simulink model "PlantaMalhaExterna_teste"  (R2018b)
settings: Solver=VariableStepAuto  StartTime=0.0  StopTime=10.0  RelTol=1e-3
undefined symbols (not defined in the file or in its folder): DiscIntNeverNeededParam
libraries: simulink x1
settings Model: Creator=lucas  LastModifiedBy=vitor
settings DataIOCC: ReturnWorkspaceOutputs=on
settings DebuggingCC: SFMachineParentedDataDiag=error

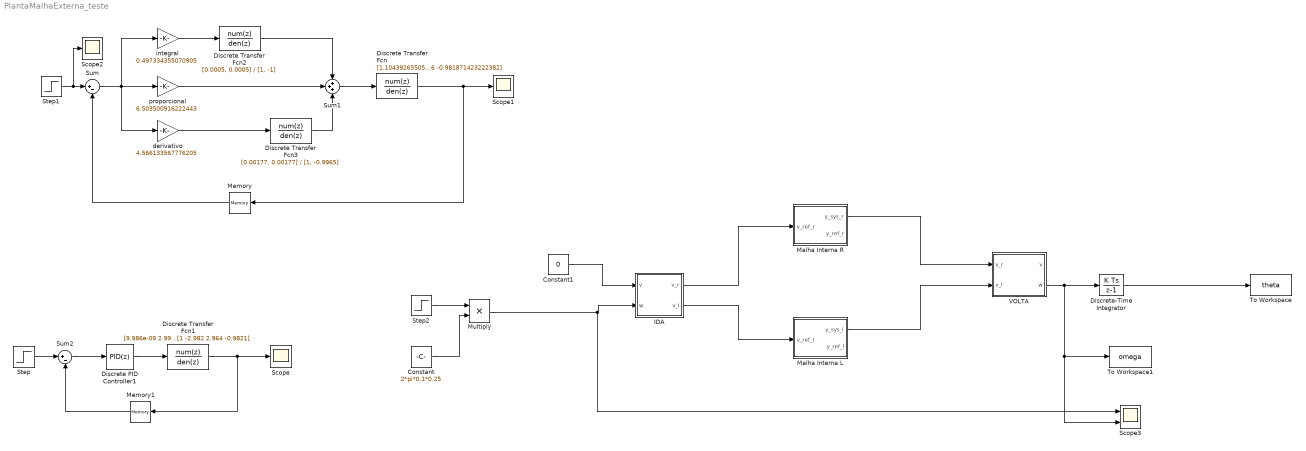
== system PlantaMalhaExterna_teste ==
  Constant : Constant  Value=2*pi*0.1*0.25
  Constant1 : Constant  Value=0
  Discrete Transfer Fcn : DiscreteTransferFcn  Numerator=[1.104392655054829e-08 3.313177965164485e-08 3.313177965164485e-08 1.104392655054829e-08]  Denominator=[1 -2.981694681338594 2.963566104560976 -0.981871423222382]  SampleTime=0.001
  Discrete Transfer Fcn1 : DiscreteTransferFcn  Numerator=[9.986e-09 2.996e-08 2.996e-08 9.986e-09]  Denominator=[1 -2.982 2.964 -0.9821]  SampleTime=0.001
  Discrete Transfer Fcn2 : DiscreteTransferFcn  Numerator=[0.0005, 0.0005]  Denominator=[1, -1]
  Discrete Transfer Fcn3 : DiscreteTransferFcn  Numerator=[0.00177, 0.00177]  Denominator=[1, -0.9965]  SampleTime=0.001
  Discrete PID Controller1 : simulink/Continuous/PID Controller  Controller=PID  Form=Parallel  TimeDomain=Discrete-time  SampleTime=0.001  IntegratorMethod=Forward Euler  FilterMethod=Forward Euler  ControllerParametersSource=internal  P=200  I=0  D=8  UseFilter=on  N=1.824  TunerSelectOption=Transfer Function Based (PID Tuner App)  InitialConditionSource=internal  InitialConditionForIntegrator=0  InitialConditionForFilter=0  DifferentiatorICPrevScaledInput=0  ExternalReset=none  TrackingMode=off  Kt=1  LimitOutput=off  UpperSaturationLimit=inf  LowerSaturationLimit=-inf  LinearizeAsGain=off  AntiWindupMode=none  Kb=1  POutMin=[]  POutMax=[]  IOutMin=[]  IOutMax=[]  DOutMin=[]  DOutMax=[]  NOutMin=[]  NOutMax=[]  SumOutMin=[]  SumOutMax=[]  SaturationOutMin=[]  SaturationOutMax=[]  PParamMin=[]  PParamMax=[]  IParamMin=[]  IParamMax=[]  DParamMin=[]  DParamMax=[]  NParamMin=[]  NParamMax=[]  KbParamMin=[]  KbParamMax=[]  KtParamMin=[]  KtParamMax=[]  KbOutMin=[]  KbOutMax=[]  KtOutMin=[]  KtOutMax=[]  IntegratorOutMin=[]  IntegratorOutMax=[]  FilterOutMin=[]  FilterOutMax=[]  SumI1OutMin=[]  SumI1OutMax=[]  SumI2OutMin=[]  SumI2OutMax=[]  SumI3OutMin=[]  SumI3OutMax=[]  SumI4OutMin=[]  SumI4OutMax=[]  SumDOutMin=[]  SumDOutMax=[]  DifferentiatorOutMin=[]  DifferentiatorOutMax=[]  FilterDiffOutCoefMin=[]  FilterDiffOutCoefMax=[]  ReciprocalOutMin=[]  ReciprocalOutMax=[]  SumDenOutMin=[]  SumDenOutMax=[]  SumNumOutMin=[]  SumNumOutMax=[]  DivideOutMin=[]  DivideOutMax=[]  IntegratorContinuousStateAttributes=''  IntegratorStateMustResolveToSignalObject=off  IntegratorRTWStateStorageClass=Auto  FilterContinuousStateAttributes=''  FilterStateMustResolveToSignalObject=off  FilterRTWStateStorageClass=Auto  ParallelPVariant=InternalParameters  IdealPVariant=Disabled  IVariant=InternalParameters  DVariant=InternalParameters  IntegratorVariant=Discrete  SatVariant=Disabled  AWVariant=Passthrough  PCopyVariant=Disabled  TRVariant=Disabled  FdbkBlocksVariant=Forward  IdealPFdbkVariant=Disabled  SatFdbkVariant=Disabled  DerivativeFilterVariant=ForwardEulerFilter  NVariant=InternalParameters  NCopyVariant=Disabled  FilterICVariant=InternalICsFilter  IntegratorICVariant=InternalICs  ExternalResetVariant=Disabled  TRSumVariant=Passthrough  SumFdbkVariant=Disabled  SumVariant=Sum_PID
  Discrete-Time Integrator : DiscreteIntegrator  SampleTime=-1  ICPrevOutput=DiscIntNeverNeededParam  ICPrevScaledInput=DiscIntNeverNeededParam
  IDA : Subsystem
  Malha Interna L : Subsystem
  Malha Interna R : Subsystem
  Memory : Memory
  Memory1 : Memory
  Multiply : Product
  Scope : Scope
  Scope1 : Scope
  Scope2 : Scope
  Scope3 : Scope  NumInputPorts=2
  Step : Step  Time=0  After=0.3  SampleTime=0.001
  Step1 : Step  Time=0  After=0.3  SampleTime=0.001
  Step2 : Step  Time=0  After=11.52  SampleTime=0.001
  Sum : Sum  Inputs=|+-
  Sum1 : Sum  Inputs=+++
  Sum2 : Sum  Inputs=|+-
  To Workspace : ToWorkspace  VariableName=theta  SaveFormat=Timeseries  SampleTime=-1
  To Workspace1 : ToWorkspace  VariableName=omega  SampleTime=-1
  VOLTA : Subsystem
  derivativo : Gain  Gain=4.566133567776205
  integral : Gain  Gain=0.497334355070905
  proporcional : Gain  Gain=6.503500916222443
  wires:
  Discrete Transfer Fcn2/1 -> Sum1/1
  proporcional/1 -> Sum1/2
  Sum1/1 -> Discrete Transfer Fcn/1
  Discrete Transfer Fcn/1 -> Scope1/1, Memory/1
  Memory/1 -> Sum/2
  Sum/1 -> derivativo/1, integral/1, proporcional/1
  Discrete PID Controller1/1 -> Discrete Transfer Fcn1/1
  Memory1/1 -> Sum2/2
  Sum2/1 -> Discrete PID Controller1/1
  Discrete Transfer Fcn1/1 -> Scope/1, Memory1/1
  Step/1 -> Sum2/1
  Discrete Transfer Fcn3/1 -> Sum1/3
  Step1/1 -> Scope2/1, Sum/1
  integral/1 -> Discrete Transfer Fcn2/1
  derivativo/1 -> Discrete Transfer Fcn3/1
  Constant1/1 -> IDA/1(v)
  Malha Interna R/1(y_sys_r) -> VOLTA/1(v_r)
  IDA/1(v_r) -> Malha Interna R/1(v_ref_r)
  Malha Interna L/1(y_sys_l) -> VOLTA/2(v_l)
  VOLTA/2(w) -> Discrete-Time Integrator/1, To Workspace1/1, Scope3/2
  IDA/2(v_l) -> Malha Interna L/1(v_ref_l)
  Discrete-Time Integrator/1 -> To Workspace/1
  Multiply/1 -> Scope3/1, IDA/2(w)
  Step2/1 -> Multiply/1
  Constant/1 -> Multiply/2

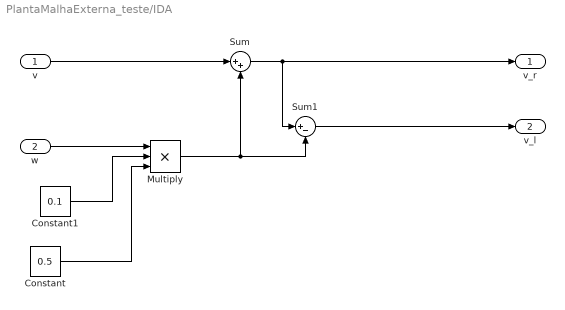
== system PlantaMalhaExterna_teste/IDA ==
  v : Inport
  w : Inport  Port=2
  Constant : Constant  Value=0.5
  Constant1 : Constant  Value=0.1
  Multiply : Product  Inputs=3
  Sum : Sum  Inputs=|++
  Sum1 : Sum  Inputs=|+-
  v_r : Outport
  v_l : Outport  Port=2
  wires:
  Multiply/1 -> Sum1/2, Sum/2
  Sum1/1 -> v_l/1
  Constant1/1 -> Multiply/2
  v/1 -> Sum/1
  w/1 -> Multiply/1
  Sum/1 -> v_r/1, Sum1/1
  Constant/1 -> Multiply/3

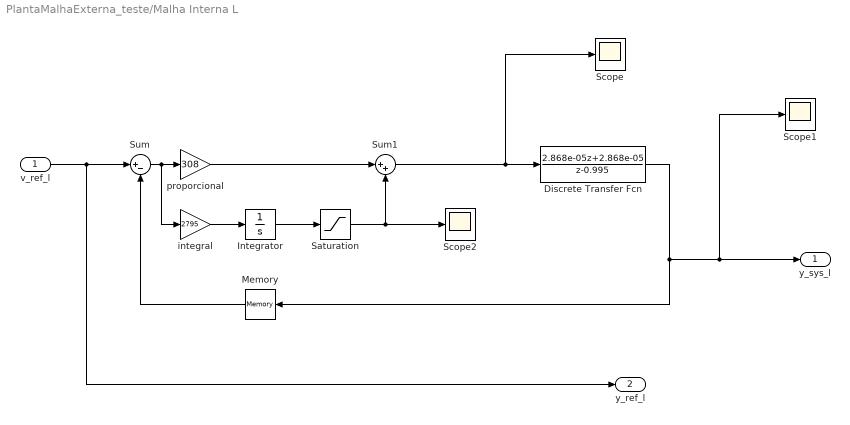
== system PlantaMalhaExterna_teste/Malha Interna L ==
  v_ref_l : Inport
  Discrete Transfer Fcn : DiscreteTransferFcn  Numerator=[2.868e-05 2.868e-05]  Denominator=[1 -0.995]  SampleTime=0.001
  Integrator : Integrator
  Memory : Memory
  Saturation : Saturate  UpperLimit=1232  LowerLimit=0
  Scope : Scope
  Scope1 : Scope
  Scope2 : Scope
  Sum : Sum  Inputs=|+-
  Sum1 : Sum  Inputs=|++
  integral : Gain  Gain=2795
  proporcional : Gain  Gain=308
  y_sys_l : Outport
  "y_ref_l " : Outport  Port=2
  wires:
  Memory/1 -> Sum/2
  Saturation/1 -> Scope2/1, Sum1/2
  proporcional/1 -> Sum1/1
  v_ref_l/1 -> "y_ref_l "/1, Sum/1
  Sum1/1 -> Scope/1, Discrete Transfer Fcn/1
  Discrete Transfer Fcn/1 -> Memory/1, y_sys_l/1, Scope1/1
  integral/1 -> Integrator/1
  Sum/1 -> integral/1, proporcional/1
  Integrator/1 -> Saturation/1

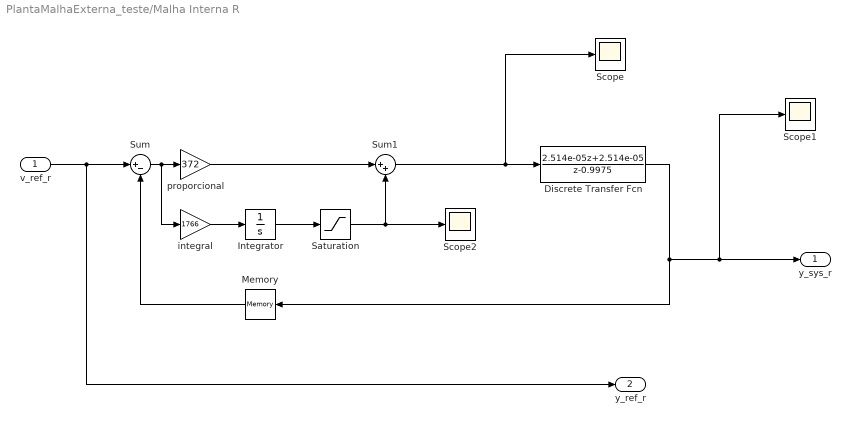
== system PlantaMalhaExterna_teste/Malha Interna R ==
  v_ref_r : Inport
  Discrete Transfer Fcn : DiscreteTransferFcn  Numerator=[2.514e-05 2.514e-05]  Denominator=[1 -0.9975]  SampleTime=0.001
  Integrator : Integrator
  Memory : Memory
  Saturation : Saturate  UpperLimit=1000  LowerLimit=0
  Scope : Scope
  Scope1 : Scope
  Scope2 : Scope
  Sum : Sum  Inputs=|+-
  Sum1 : Sum  Inputs=|++
  integral : Gain  Gain=1766
  proporcional : Gain  Gain=372
  y_sys_r : Outport
  "y_ref_r " : Outport  Port=2
  wires:
  Memory/1 -> Sum/2
  Saturation/1 -> Scope2/1, Sum1/2
  proporcional/1 -> Sum1/1
  v_ref_r/1 -> "y_ref_r "/1, Sum/1
  Sum1/1 -> Scope/1, Discrete Transfer Fcn/1
  Discrete Transfer Fcn/1 -> Memory/1, y_sys_r/1, Scope1/1
  integral/1 -> Integrator/1
  Sum/1 -> integral/1, proporcional/1
  Integrator/1 -> Saturation/1

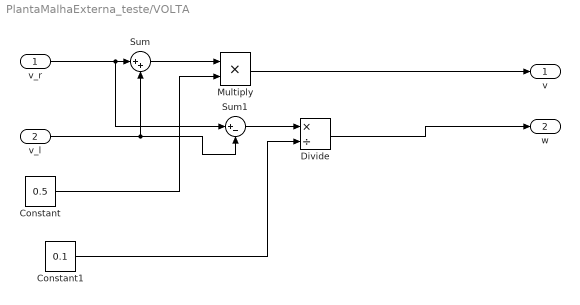
== system PlantaMalhaExterna_teste/VOLTA ==
  v_r : Inport
  v_l : Inport  Port=2
  Constant : Constant  Value=0.5
  Constant1 : Constant  Value=0.1
  Divide : Product  Inputs=*/
  Multiply : Product
  Sum : Sum  Inputs=|++
  Sum1 : Sum  Inputs=|+-
  v : Outport
  w : Outport  Port=2
  wires:
  Sum/1 -> Multiply/1
  v_l/1 -> Sum1/2, Sum/2
  Sum1/1 -> Divide/1
  v_r/1 -> Sum1/1, Sum/1
  Constant1/1 -> Divide/2
  Multiply/1 -> v/1
  Divide/1 -> w/1
  Constant/1 -> Multiply/2
